simulink model "lin_to_non-lin_model_comparison"  (R2019b)
settings: Solver=ode45  StartTime=0.0  StopTime=12  RelTol=1e-3
InitFcn:
  | addpath('generated');
  | Linearisation;
  | 
  | cst = cellulo_constants();
  | 
  | c = cst.c;
  | m = cst.m;
  | c_U=cst.c_U;
undefined symbols (not defined in the file or in its folder): Alinear, Blinear, Clinear, Dlinear, sigbuilder_block
settings Model: Creator=Hadrien  LastModifiedBy=Hadrien

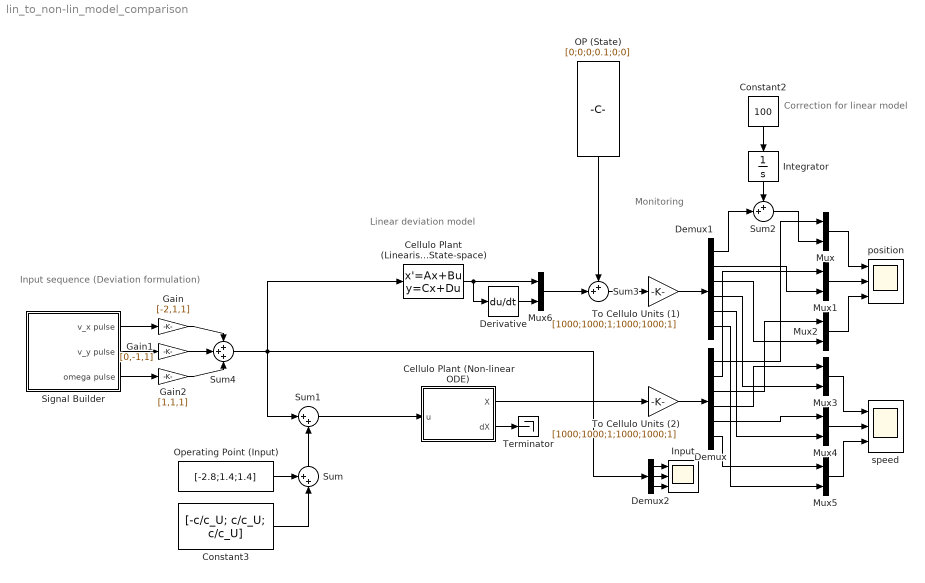
== system lin_to_non-lin_model_comparison ==
  note: Input sequence (Deviation formulation)
  note: Monitoring
  note: Linear deviation model
  note: Correction for
      | linear model
  "   OP (State)" : Constant  Value=[0;0;0;0.1;0;0]  VectorParams1D=off
  Cellulo Plant (Linearised State-space) : StateSpace  A=Alinear  B=Blinear  C=Clinear  D=Dlinear  InitialCondition=0  ContinuousStateAttributes={'x','y','th','dx','dy','dth'}
  Cellulo Plant (Non-linear ODE) : Subsystem
  Constant2 : Constant  Value=100
  Constant3 : Constant  Value="[-c/c_U;  c/c_U;  c/c_U]"  VectorParams1D=off
  Demux : Demux  Outputs=6
  Demux1 : Demux  Outputs=6
  Demux2 : Demux  Outputs=3
  Derivative : Derivative  CoefficientInTFapproximation=1
  Gain : Gain  Gain=[-2,1,1]
  Gain1 : Gain  Gain=[0,-1,1]
  Gain2 : Gain  Gain=[1,1,1]
  Input : Scope  NumInputPorts=3
  Integrator : Integrator
  Mux{,1..6} (7 alike) : Mux  Inputs=2
  Operating Point (Input) : Constant  Value=[-2.8;1.4;1.4]  VectorParams1D=off
  Signal Builder : Subsystem  Tag=STV Subsys  LoadFcn=sigbuilder_block('load');  StartFcn=sigbuilder_block('start');  StopFcn=sigbuilder_block('stop');  ClipboardFcn=sigbuilder_block('clipboard');  mask(Sigbuilder block){tuvar=[0:10]}
      mask help: Simulink:masks:SigbuilderBlock_MD
      mask init:
      | if ~strcmp(get_param(bdroot(gcbh),'SimulationStatus'),'stopped') tuvar = sigbuilder_block('maskInit'); end
      settings: CopyFcn=sigbuilder_block('copy');  DeleteFcn=sigbuilder_block('delete');  ModelCloseFcn=sigbuilder_block('modelClose');  PreSaveFcn=sigbuilder_block('preSave');  PauseFcn=sigbuilder_block('pause');  ContinueFcn=sigbuilder_block('continue');  NameChangeFcn=sigbuilder_block('namechange');  OpenFcn=sigbuilder_block('open',[437.6 199.2 550.4 400 ]);  CloseFcn=sigbuilder_block('close');
      mask Display: plot(0, 0, 100, 100,[2, 2, 32, 32, 2], [68, 8, 8, 68, 68],[32, 2], [38, 38], [32, 19, 2],[53, 60, 44], [32, 17, 17, 2],[16, 16, 31, 31]);txt = getActiveGroup(gcbh);text(2, 100, txt,'verticalAlignment', 'top');
  Sum : Sum  Inputs=++|
  Sum1 : Sum  Inputs=|++
  Sum2 : Sum  Inputs=++|
  Sum3 : Sum  Inputs=++|
  Sum4 : Sum  Inputs=+++
  Terminator : Terminator
  To Cellulo Units (1) : Gain  Gain=[1000;1000;1;1000;1000;1]
  To Cellulo Units (2) : Gain  Gain=[1000;1000;1;1000;1000;1]
  position : Scope  NumInputPorts=3
  speed : Scope  NumInputPorts=3
  wires:
  To Cellulo Units (2)/1 -> Demux/1
  Mux/1 -> position/1
  Mux1/1 -> position/2
  Mux3/1 -> speed/1
  Mux5/1 -> speed/3
  Mux4/1 -> speed/2
  To Cellulo Units (1)/1 -> Demux1/1
  Demux1/1 -> Sum2/2
  Constant2/1 -> Integrator/1
  Sum2/1 -> Mux/2
  Demux1/6 -> Mux5/2
  Demux1/5 -> Mux4/2
  Demux1/4 -> Mux3/2
  Demux1/2 -> Mux1/2
  Demux/1 -> Mux/1
  Demux/2 -> Mux1/1
  Demux/3 -> Mux2/1
  Demux/4 -> Mux3/1
  Demux/5 -> Mux4/1
  Demux/6 -> Mux5/1
  Demux1/3 -> Mux2/2
  Mux2/1 -> position/3
  Integrator/1 -> Sum2/1
  Sum1/1 -> Cellulo Plant (Non-linear ODE)/1(u)
  Sum3/1 -> To Cellulo Units (1)/1
  "   OP (State)"/1 -> Sum3/1
  Cellulo Plant (Non-linear ODE)/1(X) -> To Cellulo Units (2)/1
  Cellulo Plant (Non-linear ODE)/2(dX) -> Terminator/1
  Mux6/1 -> Sum3/2
  Derivative/1 -> Mux6/2
  Cellulo Plant (Linearised State-space)/1 -> Mux6/1, Derivative/1
  Operating Point (Input)/1 -> Sum/1
  Constant3/1 -> Sum/2
  Sum/1 -> Sum1/2
  Signal Builder/3(omega pulse) -> Gain2/1
  Signal Builder/2(v_y pulse) -> Gain1/1
  Signal Builder/1(v_x pulse) -> Gain/1
  Gain1/1 -> Sum4/2
  Gain/1 -> Sum4/1
  Gain2/1 -> Sum4/3
  Demux2/1 -> Input/1
  Demux2/2 -> Input/2
  Demux2/3 -> Input/3
  Sum4/1 -> Sum1/1, Demux2/1, Cellulo Plant (Linearised State-space)/1

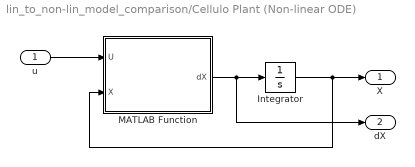
== system lin_to_non-lin_model_comparison/Cellulo Plant (Non-linear ODE) ==
  u : Inport  PortDimensions=3
  Integrator : Integrator
  MATLAB Function : MATLAB Function  TreatAsAtomicUnit=on
  X : Outport  PortDimensions=6
  dX : Outport  Port=2  PortDimensions=6
  wires:
  u/1 -> MATLAB Function/1(U)
  MATLAB Function/1(dX) -> Integrator/1, dX/1
  Integrator/1 -> X/1, MATLAB Function/2(X)

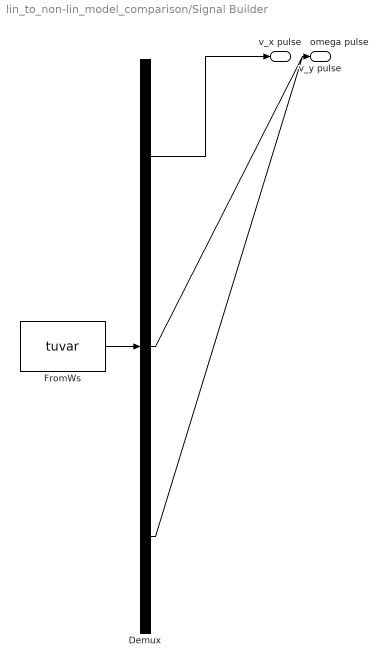
== system lin_to_non-lin_model_comparison/Signal Builder ==
  Demux : Demux  Tag=STV Demux  Outputs=3
  FromWs : FromWorkspace  Tag=STV FromWs  VariableName=tuvar  SampleTime=0
      SigBuilderData=|
      | common.afterFinalStr = 'Extrapolate'
      | common.sampleTime = 0
      | dataSet.timeRange = [0 10]
      | dataSet.name = 'Group 1'
      | sbobj.Groups.Name = 'Group 1'
      | sbobj.Groups.Signals(1).Name = 'v_x pulse'
      | sbobj.Groups.Signals(1).XData = [0 1 1 4 4 10]
      | sbobj.Groups.Signals(1).YData = [0 0 1 1 0 0]
      | sbobj.Groups.Signals(2).Name = 'v_y pulse'
      | sbobj.Groups.Signals(2).XData = [0 3 3 6 6 10]
      | sbobj.Groups.Signals(2).YData = [0 0 1 1 0 0]
      | sbobj.Groups.Signals(3).Name = 'omega pulse'
      | sbobj.Groups.Signals(3).XData = [0 7 7 9 9 10]
      | sbobj.Groups.Signals(3).YData = [0 0 1 1 0 0]
  v_x pulse : Outport  Tag=STV Outport
  v_y pulse : Outport  Tag=STV Outport  Port=2
  omega pulse : Outport  Tag=STV Outport  Port=3
  wires:
  Demux/1 -> v_x pulse/1
  FromWs/1 -> Demux/1
  Demux/2 -> v_y pulse/1
  Demux/3 -> omega pulse/1

== matlab function lin_to_non-lin_model_comparison/Cellulo Plant (Non-linear ODE)/MATLAB Function ==
  data: U input; X input; dX output
function dX = Cellulo_ODE(U,X)

x = X(1);
y = X(2);
th = X(3);
dx = X(4);
dy = X(5);
dth = X(6);
u1 = U(1);
u2 = U(2);
u3 = U(3);

M = mass();
C = coriolis();
G = gravity();
D = friction(dth,dx,dy,th,u1,u2,u3);
Q = input_forces(th);
dq = reshape(X(4:6),3,1);
ddq = M\(-C*dq - G - D + Q*[u1;u2;u3]);
dX = [dq;ddq];
